simulink subsystem "s2EMSSC"  (R2025b)
settings: Solver=VariableStepAuto  StartTime=0.0  StopTime=10.0  RelTol=1e-3
undefined symbols (not defined in the file): EM1, EM2, HVDCNeg, HVDCPos, ThrmEM1, ThrmEM2
libraries: fl_lib x14, nesl_utility_internal x10
settings Model: ModifiedByFormat=The MathWorks, Inc.  Creator=The MathWorks, Inc.  LastModifiedBy=The MathWorks, Inc.
settings RTWCC: GPUComputeCapability=3.5

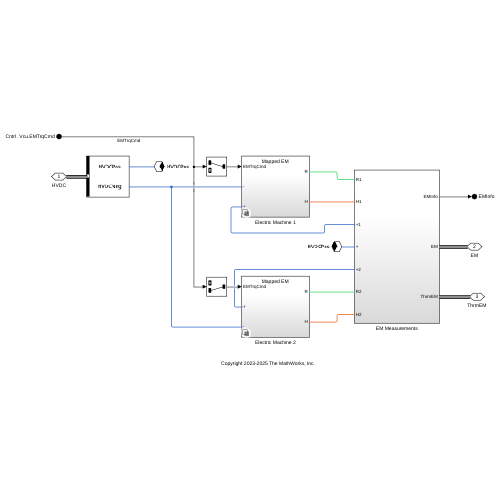
[thumbnail: Simulink's stored preview of the top-level diagram]
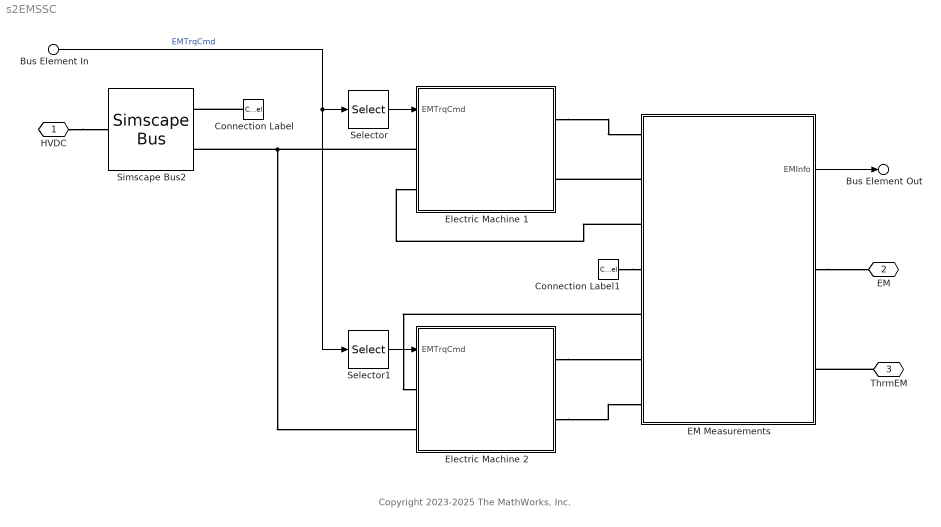
== system s2EMSSC ==
  note: Copyright 2023-2025 The MathWorks, Inc.
  Bus Element In : Inport  PortName=Cntrl  Element=Vcu.EMTrqCmd
  Connection Label : ConnectionLabel  Label=HVDCPos
  Connection Label1 : ConnectionLabel  Label=HVDCPos
  EM Measurements : Subsystem
  Electric Machine 1 : Subsystem  Variant=on  VariantControlMode=label  LabelModeActiveChoice=Mapped EM
  Electric Machine 2 : Subsystem  Variant=on  VariantControlMode=label  LabelModeActiveChoice=Mapped EM
  Selector : Selector  InputPortWidth=2  IndexOptions=Index vector (dialog)  Indices=[1]  OutputSizes=1
  Selector1 : Selector  InputPortWidth=2  IndexOptions=Index vector (dialog)  Indices=[2]  OutputSizes=1
  Simscape Bus2 : SimscapeBus  HierarchyStrings=HVDCPos;HVDCNeg
  HVDC : PMIOPort  Side=Left
  EM : PMIOPort  Port=2  Side=Right
  ThrmEM : PMIOPort  Port=3  Side=Right
  Bus Element Out : Outport  PortName=EMInfo
  wires:
  Bus Element In/1 -> Selector/1, Selector1/1  "EMTrqCmd"
  Selector/1 -> Electric Machine 1/1(EMTrqCmd)
  Selector1/1 -> Electric Machine 2/1(EMTrqCmd)
  EM Measurements/1(EMInfo) -> Bus Element Out/1
  connections:
  Electric Machine 1/LConn1 -- Electric Machine 2/LConn2 -- Simscape Bus2/LConn2
  HVDC/RConn1 -- Simscape Bus2/RConn1
  ThrmEM/RConn1 -- EM Measurements/RConn2
  EM Measurements/LConn2 -- Electric Machine 1/RConn2
  Electric Machine 1/RConn1 -- EM Measurements/LConn1
  Connection Label/LConn1 -- Simscape Bus2/LConn1
  EM Measurements/RConn1 -- EM/RConn1
  EM Measurements/LConn3 -- Electric Machine 1/LConn2
  EM Measurements/LConn5 -- Electric Machine 2/LConn1
  Electric Machine 2/RConn1 -- EM Measurements/LConn6
  Electric Machine 2/RConn2 -- EM Measurements/LConn7
  Connection Label1/LConn1 -- EM Measurements/LConn4

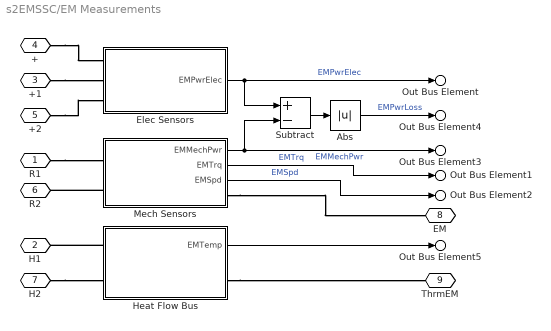
== system s2EMSSC/EM Measurements ==
  Abs : Abs  ZeroCross=off  SaturateOnIntegerOverflow=off
  Elec Sensors : Subsystem
  Heat Flow Bus : Subsystem
  Mech Sensors : Subsystem
  Subtract : Sum  Inputs=+-
  R1 : PMIOPort  Side=Left
  H1 : PMIOPort  Port=2  Side=Left
  +1 : PMIOPort  Port=3  Side=Left
  + : PMIOPort  Port=4  Side=Left
  +2 : PMIOPort  Port=5  Side=Left
  R2 : PMIOPort  Port=6  Side=Left
  H2 : PMIOPort  Port=7  Side=Left
  EM : PMIOPort  Port=8  Side=Right
  ThrmEM : PMIOPort  Port=9  Side=Right
  Out Bus Element : Outport  PortName=EMInfo  Element=EMPwrElec
  Out Bus Element1 : Outport  PortName=EMInfo  Element=EMTrq
  Out Bus Element2 : Outport  PortName=EMInfo  Element=EMSpd
  Out Bus Element3 : Outport  PortName=EMInfo  Element=EMMechPwr
  Out Bus Element4 : Outport  PortName=EMInfo  Element=EMPwrLoss
  Out Bus Element5 : Outport  PortName=EMInfo  Element=EMTemp
  wires:
  Mech Sensors/1(EMMechPwr) -> Out Bus Element3/1, Subtract/2  "EMMechPwr"
  Mech Sensors/3(EMSpd) -> Out Bus Element2/1  "EMSpd"
  Mech Sensors/2(EMTrq) -> Out Bus Element1/1  "EMTrq"
  Elec Sensors/1(EMPwrElec) -> Out Bus Element/1, Subtract/1  "EMPwrElec"
  Subtract/1 -> Abs/1
  Abs/1 -> Out Bus Element4/1  "EMPwrLoss"
  Heat Flow Bus/1(EMTemp) -> Out Bus Element5/1
  connections:
  +2/RConn1 -- Elec Sensors/LConn3
  Mech Sensors/LConn2 -- R2/RConn1
  +1/RConn1 -- Elec Sensors/LConn2
  +/RConn1 -- Elec Sensors/LConn1
  R1/RConn1 -- Mech Sensors/LConn1
  Heat Flow Bus/RConn1 -- ThrmEM/RConn1
  Mech Sensors/RConn1 -- EM/RConn1
  Heat Flow Bus/LConn1 -- H1/RConn1
  H2/RConn1 -- Heat Flow Bus/LConn2

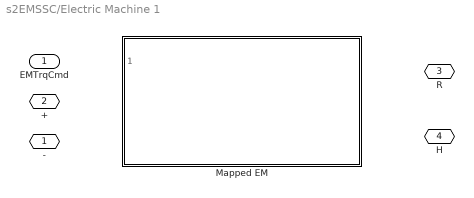
== system s2EMSSC/Electric Machine 1 ==
  EMTrqCmd : Inport
  Mapped EM : Subsystem  VariantControl=Mapped EM  ReferencedSubsystem=ElectricMachine1SSC
  - : PMIOPort  Side=Left
  + : PMIOPort  Port=2  Side=Left
  R : PMIOPort  Port=3  Side=Right
  H : PMIOPort  Port=4  Side=Right

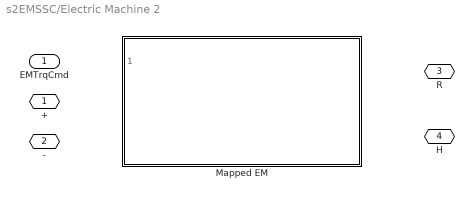
== system s2EMSSC/Electric Machine 2 ==
  EMTrqCmd : Inport
  Mapped EM : Subsystem  VariantControl=Mapped EM  ReferencedSubsystem=ElectricMachine2SSC
  + : PMIOPort  Side=Left
  - : PMIOPort  Port=2  Side=Left
  R : PMIOPort  Port=3  Side=Right
  H : PMIOPort  Port=4  Side=Right

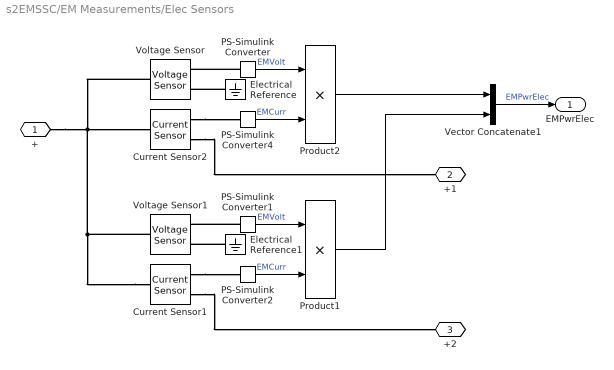
== system s2EMSSC/EM Measurements/Elec Sensors ==
  Current Sensor1 : fl_lib/Electrical/Electrical Sensors/Current Sensor
  Current Sensor2 : fl_lib/Electrical/Electrical Sensors/Current Sensor
  Electrical Reference : fl_lib/Electrical/Electrical Elements/Electrical Reference
  Electrical Reference1 : fl_lib/Electrical/Electrical Elements/Electrical Reference
  PS-Simulink Converter : nesl_utility_internal/PS-Simulink Converter  PhysicalDomain=network_engine_domain  SubClassName=ps_output  LeftPortType=input  RightPortType=output  PseudoPeriodic=off  Frequencies=[]  VectorFormat=1-D array  Unit=inherit  AffineConversion=off
  PS-Simulink Converter1 : nesl_utility_internal/PS-Simulink Converter  PhysicalDomain=network_engine_domain  SubClassName=ps_output  LeftPortType=input  RightPortType=output  PseudoPeriodic=off  Frequencies=[]  VectorFormat=1-D array  Unit=inherit  AffineConversion=off
  PS-Simulink Converter2 : nesl_utility_internal/PS-Simulink Converter  PhysicalDomain=network_engine_domain  SubClassName=ps_output  LeftPortType=input  RightPortType=output  PseudoPeriodic=off  Frequencies=[]  VectorFormat=1-D array  Unit=1  AffineConversion=off
  PS-Simulink Converter4 : nesl_utility_internal/PS-Simulink Converter  PhysicalDomain=network_engine_domain  SubClassName=ps_output  LeftPortType=input  RightPortType=output  PseudoPeriodic=off  Frequencies=[]  VectorFormat=1-D array  Unit=1  AffineConversion=off
  Product1 : Product
  Product2 : Product
  Vector Concatenate1 : Concatenate
  Voltage Sensor : fl_lib/Electrical/Electrical Sensors/Voltage Sensor
  Voltage Sensor1 : fl_lib/Electrical/Electrical Sensors/Voltage Sensor
  + : PMIOPort  Side=Left
  +1 : PMIOPort  Port=2  Side=Left
  +2 : PMIOPort  Port=3  Side=Left
  EMPwrElec : Outport
  wires:
  Product1/1 -> Vector Concatenate1/2
  Vector Concatenate1/1 -> EMPwrElec/1  "EMPwrElec"
  Product2/1 -> Vector Concatenate1/1
  PS-Simulink Converter2/1 -> Product1/2  "EMCurr"
  PS-Simulink Converter1/1 -> Product1/1  "EMVolt"
  PS-Simulink Converter/1 -> Product2/1  "EMVolt"
  PS-Simulink Converter4/1 -> Product2/2  "EMCurr"
  connections:
  Electrical Reference1/LConn1 -- Voltage Sensor1/RConn2
  Current Sensor1/RConn1 -- PS-Simulink Converter2/LConn1
  Current Sensor1/RConn2 -- +2/RConn1
  PS-Simulink Converter1/LConn1 -- Voltage Sensor1/RConn1
  PS-Simulink Converter/LConn1 -- Voltage Sensor/RConn1
  Electrical Reference/LConn1 -- Voltage Sensor/RConn2
  Current Sensor1/LConn1 -- Current Sensor2/LConn1 -- +/RConn1 -- Voltage Sensor/LConn1 -- Voltage Sensor1/LConn1
  Current Sensor2/RConn2 -- +1/RConn1
  Current Sensor2/RConn1 -- PS-Simulink Converter4/LConn1

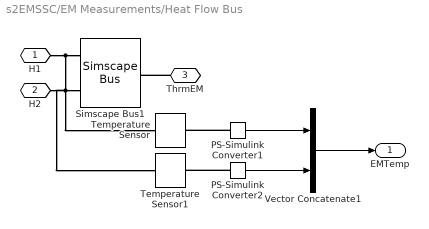
== system s2EMSSC/EM Measurements/Heat Flow Bus ==
  PS-Simulink Converter1 : nesl_utility_internal/PS-Simulink Converter  PhysicalDomain=network_engine_domain  SubClassName=ps_output  LeftPortType=input  RightPortType=output  PseudoPeriodic=off  Frequencies=[]  VectorFormat=1-D array  Unit=K  AffineConversion=on
  PS-Simulink Converter2 : nesl_utility_internal/PS-Simulink Converter  PhysicalDomain=network_engine_domain  SubClassName=ps_output  LeftPortType=input  RightPortType=output  PseudoPeriodic=off  Frequencies=[]  VectorFormat=1-D array  Unit=K  AffineConversion=on
  Simscape Bus1 : SimscapeBus  HierarchyStrings=ThrmEM1;ThrmEM2
  Temperature Sensor : fl_lib/Thermal/Thermal Sensors/Temperature Sensor  temperature_measure=foundation.enum.MeasurementReference.absolute
      settings: InternalSimscapePortConfiguration="{\"Bottom\":[],\"Left\":[{\"id\":\"A\",\"label\":\"A\",\"type\":\"foundation.thermal.thermal\"}],\"Right\":[{\"id\":\"T\",\"label\":\"T\",\"type\":\"output\"}],\"Top\":[]}"
  Temperature Sensor1 : fl_lib/Thermal/Thermal Sensors/Temperature Sensor  temperature_measure=foundation.enum.MeasurementReference.absolute
      settings: InternalSimscapePortConfiguration="{\"Bottom\":[],\"Left\":[{\"id\":\"A\",\"label\":\"A\",\"type\":\"foundation.thermal.thermal\"}],\"Right\":[{\"id\":\"T\",\"label\":\"T\",\"type\":\"output\"}],\"Top\":[]}"
  Vector Concatenate1 : Concatenate
  H1 : PMIOPort  Side=Left
  H2 : PMIOPort  Port=2  Side=Left
  ThrmEM : PMIOPort  Port=3  Side=Right
  EMTemp : Outport
  wires:
  PS-Simulink Converter1/1 -> Vector Concatenate1/1
  PS-Simulink Converter2/1 -> Vector Concatenate1/2
  Vector Concatenate1/1 -> EMTemp/1
  connections:
  H1/RConn1 -- Temperature Sensor/LConn1 -- Simscape Bus1/LConn1
  H2/RConn1 -- Temperature Sensor1/LConn1 -- Simscape Bus1/LConn2
  ThrmEM/RConn1 -- Simscape Bus1/RConn1
  PS-Simulink Converter1/LConn1 -- Temperature Sensor/RConn1
  PS-Simulink Converter2/LConn1 -- Temperature Sensor1/RConn1

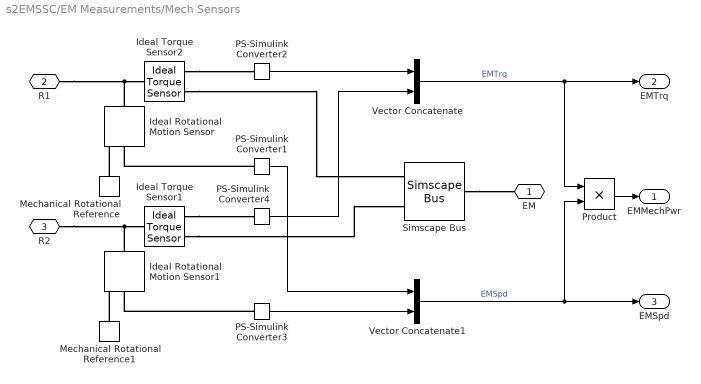
== system s2EMSSC/EM Measurements/Mech Sensors ==
  Ideal Rotational Motion Sensor : fl_lib/Mechanical/Mechanical Sensors/Ideal Rotational Motion Sensor  reference=foundation.enum.MeasurementReference.difference  acceleration_port=false  velocity_port=true  position_port=true  wrap_angle=false  offset=0 rad
  Ideal Rotational Motion Sensor1 : fl_lib/Mechanical/Mechanical Sensors/Ideal Rotational Motion Sensor  reference=foundation.enum.MeasurementReference.difference  acceleration_port=false  velocity_port=true  position_port=true  wrap_angle=false  offset=0 rad
  Ideal Torque Sensor1 : fl_lib/Mechanical/Mechanical Sensors/Ideal Torque Sensor
  Ideal Torque Sensor2 : fl_lib/Mechanical/Mechanical Sensors/Ideal Torque Sensor
  Mechanical Rotational Reference : fl_lib/Mechanical/Rotational Elements/Mechanical Rotational Reference
  Mechanical Rotational Reference1 : fl_lib/Mechanical/Rotational Elements/Mechanical Rotational Reference
  PS-Simulink Converter1 : nesl_utility_internal/PS-Simulink Converter  PhysicalDomain=network_engine_domain  SubClassName=ps_output  LeftPortType=input  RightPortType=output  PseudoPeriodic=off  Frequencies=[]  VectorFormat=1-D array  Unit=rad/s  AffineConversion=off
  PS-Simulink Converter2 : nesl_utility_internal/PS-Simulink Converter  PhysicalDomain=network_engine_domain  SubClassName=ps_output  LeftPortType=input  RightPortType=output  PseudoPeriodic=off  Frequencies=[]  VectorFormat=1-D array  Unit=1  AffineConversion=off
  PS-Simulink Converter3 : nesl_utility_internal/PS-Simulink Converter  PhysicalDomain=network_engine_domain  SubClassName=ps_output  LeftPortType=input  RightPortType=output  PseudoPeriodic=off  Frequencies=[]  VectorFormat=1-D array  Unit=rad/s  AffineConversion=off
  PS-Simulink Converter4 : nesl_utility_internal/PS-Simulink Converter  PhysicalDomain=network_engine_domain  SubClassName=ps_output  LeftPortType=input  RightPortType=output  PseudoPeriodic=off  Frequencies=[]  VectorFormat=1-D array  Unit=1  AffineConversion=off
  Product : Product
  Simscape Bus : SimscapeBus  HierarchyStrings=EM1;EM2
  Vector Concatenate : Concatenate
  Vector Concatenate1 : Concatenate
  EM : PMIOPort  Side=Right
  R1 : PMIOPort  Port=2  Side=Left
  R2 : PMIOPort  Port=3  Side=Left
  EMMechPwr : Outport
  EMTrq : Outport  Port=2
  EMSpd : Outport  Port=3
  wires:
  Product/1 -> EMMechPwr/1
  Vector Concatenate1/1 -> EMSpd/1, Product/2  "EMSpd"
  Vector Concatenate/1 -> EMTrq/1, Product/1  "EMTrq"
  PS-Simulink Converter3/1 -> Vector Concatenate1/2
  PS-Simulink Converter4/1 -> Vector Concatenate/2
  PS-Simulink Converter1/1 -> Vector Concatenate1/1
  PS-Simulink Converter2/1 -> Vector Concatenate/1
  connections:
  Simscape Bus/RConn1 -- EM/RConn1
  PS-Simulink Converter3/LConn1 -- Ideal Rotational Motion Sensor1/RConn2
  Ideal Torque Sensor1/RConn1 -- Simscape Bus/LConn2
  Mechanical Rotational Reference1/LConn1 -- Ideal Rotational Motion Sensor1/RConn1
  Ideal Torque Sensor1/RConn2 -- PS-Simulink Converter4/LConn1
  Ideal Rotational Motion Sensor1/LConn1 -- Ideal Torque Sensor1/LConn1 -- R2/RConn1
  PS-Simulink Converter1/LConn1 -- Ideal Rotational Motion Sensor/RConn2
  Mechanical Rotational Reference/LConn1 -- Ideal Rotational Motion Sensor/RConn1
  Ideal Torque Sensor2/RConn1 -- Simscape Bus/LConn1
  Ideal Rotational Motion Sensor/LConn1 -- R1/RConn1 -- Ideal Torque Sensor2/LConn1
  Ideal Torque Sensor2/RConn2 -- PS-Simulink Converter2/LConn1
